simulink model "gm_FFTHDLOptimizedExample_Burst"  (R2022a)
settings: Solver=FixedStepDiscrete  StartTime=0.0  StopTime=48*FFTLength  RelTol=1e-3
InitFcn:
  | FFTLength = 2^9;
  | ValidPattern = 1;
  | Fs = 1*2e6;
libraries: dsphdlxfrm2 x1, dspmathops x1
settings Model: Creator=The MathWorks, Inc.  LastModifiedBy=dbkomma
settings SolverCC: AlgebraicLoopSolver=TrustRegion  MaxZcPerStep=1
settings DataIOCC: SaveOutput=off  SaveTime=off  ReturnWorkspaceOutputs=off
settings OptimizationCC: BlockReduction=off  ConditionallyExecuteInputs=off  DefaultParameterBehavior=Inlined
settings DebuggingCC: AlgebraicLoopMsg=error  InheritedTsInSrcMsg=none  SingleTaskRateTransMsg=error  UnconnectedInputMsg=warning  UnconnectedOutputMsg=warning  UnconnectedLineMsg=warning  SFMachineParentedDataDiag=warning  ArithmeticOperatorsInVariantConditions=warning
settings HardwareCC: ProdBitPerPointer=32  ProdBitPerSizeT=32  ProdBitPerPtrDiffT=32  ProdLargestAtomicFloat=None  ProdIntDivRoundTo=Undefined  ProdEndianess=Unspecified  ProdWordSize=32  ProdHWDeviceType=ASIC/FPGA->ASIC/FPGA  ProdEqTarget=off
settings SFSimCC: SimUseLocalCustomCode=off  CustomCodeUndefinedFunction=UseInterfaceOnly
settings RTWCC: RTWUseLocalCustomCode=off  DLArmComputeVersion=19.05
settings CodeAppCC: StateflowObjectComments=on

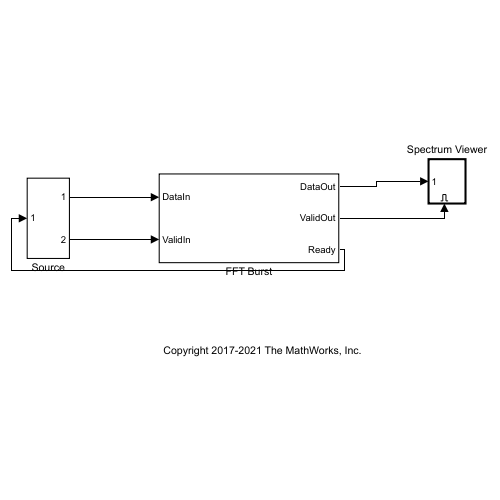
[thumbnail: Simulink's stored preview of the top-level diagram]
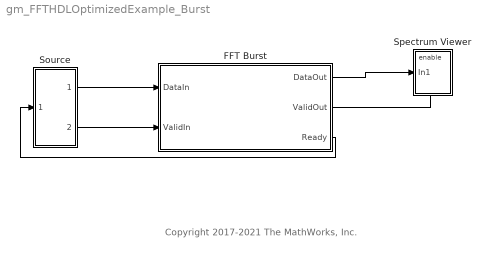
== system gm_FFTHDLOptimizedExample_Burst ==
  note: Copyright 2017-2021 The MathWorks, Inc.
  FFT Burst : Subsystem
  Source : Subsystem
  Spectrum Viewer : Subsystem
  wires:
  FFT Burst/2(ValidOut) -> Spectrum Viewer/Enable
  Source/2(Out2) -> FFT Burst/2(ValidIn)
  Source/1(Out1) -> FFT Burst/1(DataIn)
  FFT Burst/3(Ready) -> Source/1(In1)
  FFT Burst/1(DataOut) -> Spectrum Viewer/1(In1)

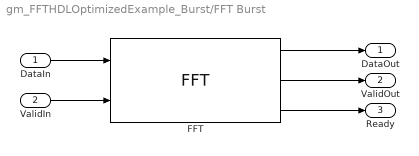
== system gm_FFTHDLOptimizedExample_Burst/FFT Burst ==
  DataIn : Inport
  ValidIn : Inport  Port=2
  FFT : dsphdlxfrm2/FFT  FFTLength=FFTLength  Architecture=Burst Radix 2  ComplexMultiplication=Use 4 multipliers and 2 adders  BitReversedOutput=on  BitReversedInput=off  Normalize=off  SimulateUsing=Code generation  RoundingMethod=Floor  ResetInputPort=off  StartOutputPort=off  EndOutputPort=off
      settings: SourceProductBaseCode=HS
  DataOut : Outport  VectorParamsAs1DForOutWhenUnconnected=off
  ValidOut : Outport  Port=2  VectorParamsAs1DForOutWhenUnconnected=off
  Ready : Outport  Port=3  VectorParamsAs1DForOutWhenUnconnected=off
  wires:
  FFT/2 -> ValidOut/1
  FFT/3 -> Ready/1
  FFT/1 -> DataOut/1
  ValidIn/1 -> FFT/2
  DataIn/1 -> FFT/1

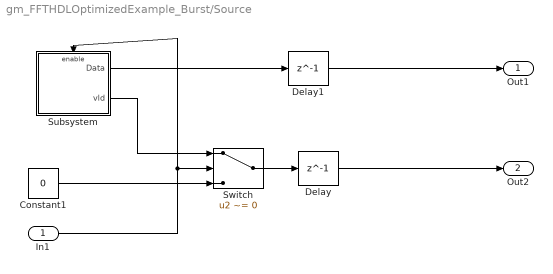
== system gm_FFTHDLOptimizedExample_Burst/Source ==
  In1 : Inport
  Constant1 : Constant  Value=0  OutDataTypeStr=boolean  SampleTime=-1
  Delay : Delay  DelayLength=1
  Delay1 : Delay  DelayLength=1
  Subsystem : Subsystem
  Switch : Switch  Criteria=u2 ~= 0  Threshold=1  SaturateOnIntegerOverflow=off  InputSameDT=off
  Out1 : Outport  VectorParamsAs1DForOutWhenUnconnected=off
  Out2 : Outport  Port=2  VectorParamsAs1DForOutWhenUnconnected=off
  wires:
  Switch/1 -> Delay/1
  Subsystem/1(Data) -> Delay1/1
  Delay1/1 -> Out1/1
  Delay/1 -> Out2/1
  In1/1 -> Switch/2, Subsystem/Enable
  Subsystem/2(vld) -> Switch/1
  Constant1/1 -> Switch/3

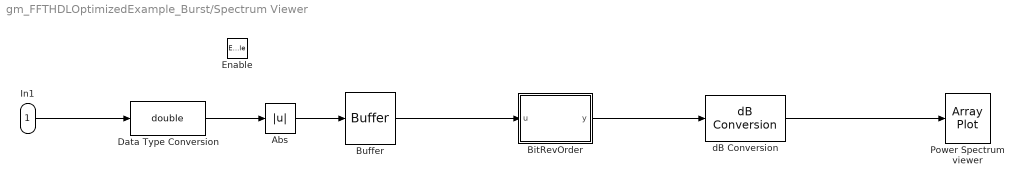
== system gm_FFTHDLOptimizedExample_Burst/Spectrum Viewer ==
  In1 : Inport
  Enable : EnablePort
  Abs : Abs  SaturateOnIntegerOverflow=off
  BitRevOrder : MATLAB Function  TreatAsAtomicUnit=on
  Buffer : Buffer  N=FFTLength  OutputFrames=off
  Data Type Conversion : DataTypeConversion  OutDataTypeStr=double  SaturateOnIntegerOverflow=off  RndMeth=Floor
  Power Spectrum viewer : ArrayPlot  WindowPosition=[1154.000000,405.000000,751.000000,427.000000,]  ScopeFrameLocation=window  SampleIncrement=Fs/FFTLength  PlotType=Stairs  AxesScaling=Manual  Title=Power Spectrum  XLabel=Frequency  YLabel=dBm  YLimits=[-60,60]  DefaultConfigurationName=dsp.scopes.ArrayPlotBlockSpecification
  dB Conversion : dspmathops/dB Conversion  dBtype=dB  intype=Amplitude  R=1  fuzz=on
  wires:
  In1/1 -> Data Type Conversion/1
  Abs/1 -> Buffer/1
  Data Type Conversion/1 -> Abs/1
  dB Conversion/1 -> Power Spectrum viewer/1
  BitRevOrder/1(y) -> dB Conversion/1
  Buffer/1 -> BitRevOrder/1(u)

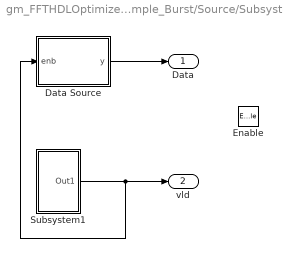
== system gm_FFTHDLOptimizedExample_Burst/Source/Subsystem ==
  Enable : EnablePort
  Data Source : MATLAB Function  TreatAsAtomicUnit=on
  Subsystem1 : Subsystem
  Data : Outport  VectorParamsAs1DForOutWhenUnconnected=off
  vld : Outport  Port=2  VectorParamsAs1DForOutWhenUnconnected=off
  wires:
  Subsystem1/1(Out1) -> vld/1, Data Source/1(enb)
  Data Source/1(y) -> Data/1

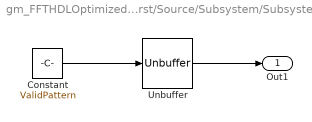
== system gm_FFTHDLOptimizedExample_Burst/Source/Subsystem/Subsystem1 ==
  Constant : Constant  Value=ValidPattern  OutDataTypeStr=boolean  SampleTime=-1
  Unbuffer : Unbuffer
  Out1 : Outport  VectorParamsAs1DForOutWhenUnconnected=off
  wires:
  Unbuffer/1 -> Out1/1
  Constant/1 -> Unbuffer/1

== matlab function gm_FFTHDLOptimizedExample_Burst/Source/Subsystem/Data Source ==
  settings: updateMethod=DISCRETE  sampleTime=1
  data: enb input; y output size=1; Fs parameter
function y = fcn(enb, Fs)
persistent sinegen1 sinegen2

noiseVar   = 1e-12;
if isempty(sinegen1)
    sinegen1 = dsp.SineWave('Amplitude', 1, 'Frequency',200000, 'SampleRate',Fs);
    sinegen2 = dsp.SineWave('Amplitude', 2, 'Frequency',250000, 'SampleRate',Fs);
end

if enb  
    y = complex(fi(sinegen1() + sinegen2() + sqrt(noiseVar)*randn(1,1), 1, 16, 13));
else
    y = complex(fi(0, 1, 16, 13));
end

== matlab function gm_FFTHDLOptimizedExample_Burst/Spectrum Viewer/BitRevOrder ==
  data: u input; y output size=[FFTLength, 1]
function y = fcn(u)

%#codegen

y = bitrevorder(u);
